simulink model "w1p2"  (R2020a)
settings: Solver=VariableStepAuto  StartTime=0.0  StopTime=100  RelTol=1e-3
values from neighbouring files (symbols this model uses):
  B = 7500    [w1p2.mat]
  K1 = 32000    [w1p2.mat]
  K2 = 65000    [w1p2.mat]
  M1 = 500    [w1p2.mat]
  M2 = 15    [w1p2.mat]
settings Model: Creator=Shubham  LastModifiedBy=Shubham

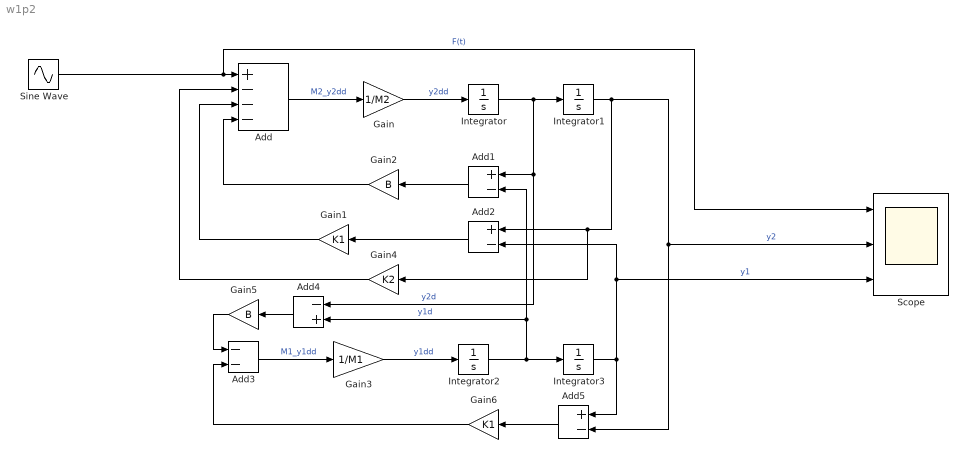
== system w1p2 ==
  Add : Sum  Inputs=+---
  Add1 : Sum  Inputs=+-
  Add2 : Sum  Inputs=+-
  Add3 : Sum  Inputs=--
  Add4 : Sum  Inputs=-+
  Add5 : Sum  Inputs=+-
  Gain : Gain  Gain=1/M2
  Gain1 : Gain  Gain=K1
  Gain2 : Gain  Gain=B
  Gain3 : Gain  Gain=1/M1
  Gain4 : Gain  Gain=K2
  Gain5 : Gain  Gain=B
  Gain6 : Gain  Gain=K1
  Integrator{,1..3} (4 alike) : Integrator
  Scope : Scope  NumInputPorts=3
  Sine Wave : Sin  Frequency=0.1  SampleTime=0
  wires:
  Add/1 -> Gain/1  "M2_y2dd"
  Gain/1 -> Integrator/1  "y2dd"
  Integrator/1 -> Add4/1, Add1/1, Integrator1/1  "y2d"
  Sine Wave/1 -> Scope/1, Add/1  "F(t)"
  Add1/1 -> Gain2/1
  Integrator2/1 -> Add4/2, Add1/2, Integrator3/1  "y1d"
  Gain3/1 -> Integrator2/1  "y1dd"
  Gain2/1 -> Add/4
  Integrator3/1 -> Add2/2, Scope/3, Add5/1  "y1"
  Add2/1 -> Gain1/1
  Gain1/1 -> Add/3
  Gain4/1 -> Add/2
  Integrator1/1 -> Gain4/1, Add2/1, Add5/2, Scope/2  "y2"
  Add3/1 -> Gain3/1  "M1_y1dd"
  Add4/1 -> Gain5/1
  Gain5/1 -> Add3/1
  Add5/1 -> Gain6/1
  Gain6/1 -> Add3/2
